simulink model "recursive_arx"  (R2015a)
settings: Solver=ode45  SolverMode=SingleTasking  StartTime=0.0  StopTime=50  RelTol=1e-3
undefined symbols (not defined in the file): den, num, R, S, T
settings Model: CovMetricSettings=dwe  CovHtmlReporting=off  covSaveCumulativeToWorkspaceVar=off  CovSaveSingleToWorkspaceVar=off  CovExternalEMLEnable=on  Creator=Carlos Henrique  LastModifiedBy=controle
settings DataIOCC: LimitDataPoints=off  SaveFormat=StructureWithTime
settings DebuggingCC: SFUnexpectedBacktrackingDiag=error  SFNoUnconditionalDefaultTransitionDiag=error
settings HardwareCC: ProdBitPerPointer=64  ProdLargestAtomicFloat=Float  ProdIntDivRoundTo=Zero  ProdEndianess=LittleEndian  ProdHWDeviceType=Specified
settings ModelReferenceCC: PropagateSignalLabelsOutOfModel=on
settings SFSimCC: SimUseLocalCustomCode=on
settings RTWCC: RTWUseLocalCustomCode=on
settings GRTTargetCC: TargetLangStandard=C99 (ISO)  GeneratePreprocessorConditionals=Use local settings

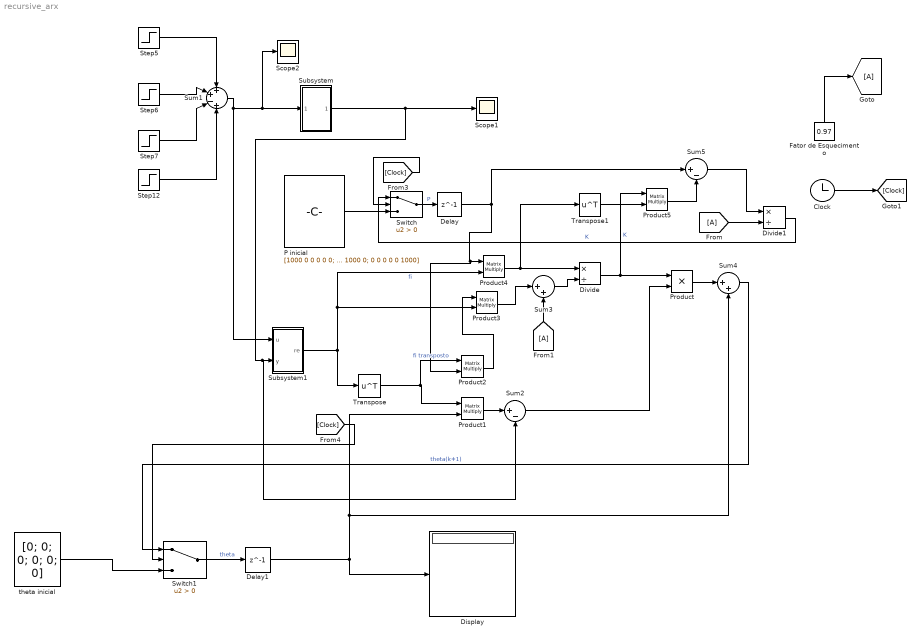
== system recursive_arx ==
  Clock : Clock
  Delay : Delay  DelayLength=1  InitialCondition=0  SampleTime=0.1
  Delay1 : Delay  DelayLength=1  InitialCondition=0  SampleTime=0.1
  Display : Display
  Divide : Product  Inputs=*/
  Divide1 : Product  Inputs=*/
  "Fator de Esquecimento " : Constant  Value=0.97
  P inicial : Constant  Value=[1000 0 0 0 0 0; 0 1000 0 0 0 0; 0 0 1000 0 0 0; 0 0 0 1000 0 0; 0 0 0 0 1000 0; 0 0 0 0 0 1000]
  Product : Product
  Product{1..5} (5 alike) : Product  Multiplication=Matrix(*)
  Scope1 : Scope
      settings: YMin=-0.1368  YMax=1.23123  SaveName=ScopeData2
  Scope2 : Scope
      settings: YMin=-0.1368  YMax=1.23123
  Step12 : Step  Time=30  SampleTime=0
  Step5 : Step  Time=0  SampleTime=0
  Step6 : Step  Time=10  After=3  SampleTime=0
  Step7 : Step  Time=20  After=2  SampleTime=0
  Subsystem : Subsystem
  Subsystem1 : Subsystem
  Sum1 : Sum  Inputs=++-+
  Sum2 : Sum  Inputs=|+-
  Sum3 : Sum  Inputs=|++
  Sum4 : Sum  Inputs=|++
  Sum5 : Sum  Inputs=|+-
  Switch : Switch  Criteria=u2 > Threshold
  Switch1 : Switch  Criteria=u2 > Threshold
  Transpose : Math  Operator=transpose  SaturateOnIntegerOverflow=on
  Transpose1 : Math  Operator=transpose  SaturateOnIntegerOverflow=on
  "theta inicial " : Constant  Value=[0; 0; 0; 0; 0; 0]
  wires:
  Step12/1 -> Sum1/4
  Step7/1 -> Sum1/3
  Step6/1 -> Sum1/2
  Step5/1 -> Sum1/1
  Sum1/1 -> Subsystem1/1(u), Scope2/1, Subsystem/1(In1)
  Subsystem/1(Out1) -> Sum2/2, Subsystem1/2(y), Scope1/1
  Subsystem1/1(re) -> Transpose/1, Product4/2, Product3/2  "fi"
  Transpose/1 -> Product2/1, Product1/1  "fi transposto"
  Product1/1 -> Sum2/1
  Sum2/1 -> Product/2
  Product4/1 -> Transpose1/1, Divide/1
  [A] -> Sum3/2
  Sum3/1 -> Divide/2
  Product3/1 -> Sum3/1
  Product2/1 -> Product3/1
  Divide/1 -> Product5/1, Product/1  "K"
  Product/1 -> Sum4/1
  "Fator de Esquecimento "/1 -> [A]
  [A] -> Divide1/2
  Transpose1/1 -> Product5/2
  Product5/1 -> Sum5/2
  Sum5/1 -> Divide1/1
  Clock/1 -> [Clock]
  [Clock] -> Switch/2
  [Clock] -> Switch1/2
  Divide1/1 -> Switch/1  "K"
  P inicial/1 -> Switch/3
  Sum4/1 -> Switch1/1  "theta(k+1)"
  "theta inicial "/1 -> Switch1/3
  Switch/1 -> Delay/1  "P"
  Delay/1 -> Product2/2, Product4/1, Sum5/1
  Switch1/1 -> Delay1/1  "theta"
  Delay1/1 -> Sum4/2, Product1/2, Display/1

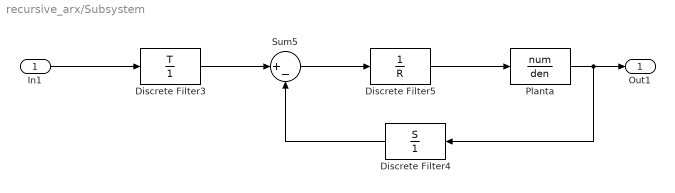
== system recursive_arx/Subsystem ==
  In1 : Inport
  Discrete Filter3 : DiscreteFilter  Numerator=T  Denominator=1  SampleTime=0.1
  Discrete Filter4 : DiscreteFilter  Numerator=S  Denominator=1  SampleTime=0.1
  Discrete Filter5 : DiscreteFilter  Numerator=1  Denominator=R  SampleTime=0.1
  "Planta " : DiscreteFilter  Numerator=num  Denominator=den  SampleTime=0.1
  Sum5 : Sum  Inputs=|+-
  Out1 : Outport
  wires:
  Discrete Filter5/1 -> "Planta "/1
  Sum5/1 -> Discrete Filter5/1
  Discrete Filter3/1 -> Sum5/1
  In1/1 -> Discrete Filter3/1
  Discrete Filter4/1 -> Sum5/2
  "Planta "/1 -> Out1/1, Discrete Filter4/1

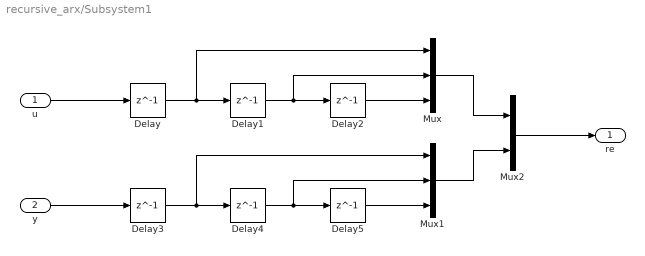
== system recursive_arx/Subsystem1 ==
  u : Inport
  y : Inport  Port=2
  Delay{,1..5} (6 alike) : Delay  DelayLength=1  InitialCondition=0  SampleTime=0.1
  Mux : Mux  Inputs=3
  Mux1 : Mux  Inputs=3
  Mux2 : Mux  Inputs=2
  re : Outport
  wires:
  Delay4/1 -> Mux1/2, Delay5/1
  u/1 -> Delay/1
  Delay5/1 -> Mux1/3
  Delay/1 -> Mux/1, Delay1/1
  Mux1/1 -> Mux2/2
  Delay1/1 -> Mux/2, Delay2/1
  Mux/1 -> Mux2/1
  Mux2/1 -> re/1
  Delay3/1 -> Mux1/1, Delay4/1
  Delay2/1 -> Mux/3
  y/1 -> Delay3/1
